simulink model "Model_14Bus_Microgrid_paper_Latam"  (R2022b)
settings: Solver=VariableStepAuto  StartTime=0.0  StopTime=0.5  MaxStep=1e-2  RelTol=1e-3
InitFcn:
  | Set_parameters_R2018
StopFcn:
  | %Save_Data;
  | %Graphics_mod;
values from neighbouring files (symbols this model uses):
  Clink = Ceq*2    (= 0.217013888889)    [Set_parameters.m]
  dis1 = 0.15    [Set_parameters.m]
  dis10 = 6    [Set_parameters.m]
  dis11 = 3    [Set_parameters.m]
  dis12 = 6    [Set_parameters.m]
  dis13 = 3    [Set_parameters.m]
  dis14 = 2    [Set_parameters.m]
  dis2 = 0.2    [Set_parameters.m]
  dis3 = 0.15    [Set_parameters.m]
  dis4 = 0.4    [Set_parameters.m]
  dis5 = 0.4    [Set_parameters.m]
  dis6 = 0.4    [Set_parameters.m]
  dis7 = 0.1    [Set_parameters.m]
  dis8 = 2    [Set_parameters.m]
  dis9 = 6    [Set_parameters.m]
  Fc = 33 * Fnom    (= 1980)    [Set_parameters.m]
  Fnom = 60    [Set_parameters.m]
  Increment_MPPT = 0.01    [Set_parameters.m]
  Ki_Ireg = 20    [Set_parameters.m]
  Ki_VDCreg = 400    [Set_parameters.m]
  Kp_Ireg = 0.3    [Set_parameters.m]
  Kp_VDCreg = 2    [Set_parameters.m]
  LimitL_Ireg = -1.5    [Set_parameters.m]
  LimitL_VDCreg = -1.5    [Set_parameters.m]
  Limits_MPPT = [ 583 357 ]    [Set_parameters.m]
  LimitU_Ireg = 1.5    [Set_parameters.m]
  LimitU_VDCreg = 1.5    [Set_parameters.m]
  P_Load_2 = S_Load_2* PF_Load_2    (= 36000)    [Set_parameters.m]
  P_Load_3 = S_Load_3* PF_Load_3    (= 25500)    [Set_parameters.m]
  Pnom = 1e6    (= 1000000)    [Set_parameters.m]
  Pnom_T1 = 1.5e6    (= 1500000)    [Set_parameters.m]
  Pnom_T2 = 1.5e6    (= 1500000)    [Set_parameters.m]
  Pnom_T3 = 4e6    (= 4000000)    [Set_parameters.m]
  Pnom_xfo = Pnom    (= 1000000)    [Set_parameters.m]
  Ql_Load_2 = S_Load_2 * sin(acos(PF_Load_2))    [Set_parameters.m]
  Ql_Load_3 = S_Load_3 * sin(acos(PF_Load_3))    [Set_parameters.m]
  R_Load_9 = (Vnom_prim * 1.35)^2 / P_Load_9    (= 1084.6153125)    [Set_parameters.m]
  R_Load_DC = Vnom_DC^2/ P_Load_DC    (= 45)    [Set_parameters.m]
  Rl = 0.394    [Set_parameters.m]
  Rls = 0.198    [Set_parameters.m]
  Ts = Ts_Power    (= 5.05050505051e-06)    [Set_parameters.m]
  Ts_Control = 10*Ts_Power    (= 5.05050505051e-05)    [Set_parameters.m]
  Ts_Power = 1/(33*Fnom)/100    (= 5.05050505051e-06)    [Set_parameters.m]
  V1_LL_T3 = 69e3    (= 69000)    [Set_parameters.m]
  Vf = 0    [Set_parameters.m]
  Vfd = 0    [Set_parameters.m]
  Vnom_dc = 480    [Set_parameters.m]
  Vnom_Diesel = 2.4e3    (= 2400)    [Set_parameters.m]
  Vnom_prim = 13.8e3    (= 13800)    [Set_parameters.m]
  Vnom_sec = 220    [Set_parameters.m]
  Vnom_ter_AC_DC = 150    [Set_parameters.m]
  Xl = 0.1168    [Set_parameters.m]
  Xls = 0.1089    [Set_parameters.m]
undefined symbols (not defined in the file or in its folder): D1, Delta, DiscIntNeverNeededParam, Hydride, Ion, level, Lithium, max_min, Metal, Nickel, RL, RLff, sigbuilder_block
libraries: spsRMSLib x73, powerlib_extras x53, spsCurrentMeasurementLib x47, spsTHDLib x26, spsThreePhaseVIMeasurementLib x25, spsVoltageMeasurementLib x23, spsSeriesRLCBranchLib x21, spsThreePhaseSeriesRLCBranchLib x21, spsIGBTDiodeLib x15, spsThreePhaseBreakerLib x14, spsPowerLib x14, spsThreePhaseTransformerTwoWindingsLib x12
(part 3 of 10)

== system Model_14Bus_Microgrid_paper_Latam/Line 10 (6km) ==
  Bus_14 11 : Subsystem  Commented=on
  Goto30 : Goto  Commented=on  GotoTag=Ib_L10  TagVisibility=global
  Goto31 : Goto  Commented=on  GotoTag=Ic_L10  TagVisibility=global
  Goto32 : Goto  Commented=on  GotoTag=Ia_L10  TagVisibility=global
  Ia_L10 : spsCurrentMeasurementLib/Current Measurement  PhasorSimulation=off  OutputType=Complex  PSBequivalent=0
  Ib_L10 : spsCurrentMeasurementLib/Current Measurement  PhasorSimulation=off  OutputType=Complex  PSBequivalent=0
  Ic_L10 : spsCurrentMeasurementLib/Current Measurement  PhasorSimulation=off  OutputType=Complex  PSBequivalent=0
  Line10 6km : spsThreePhaseSeriesRLCBranchLib/Three-Phase Series RLC Branch  LConnTagsString=A|B|C  RConnTagsString=A|B|C  BranchType=RL  Resistance=Rl * dis10  Inductance=Xl/377 * dis10  Capacitance=1e-6  Measurements=None
  a : PMIOPort  Side=Right
  b : PMIOPort  Port=2  Side=Right
  c : PMIOPort  Port=3  Side=Right
  A : PMIOPort  Port=4  Side=Left
  B : PMIOPort  Port=5  Side=Left
  C : PMIOPort  Port=6  Side=Left
  wires:
  Ia_L10/1 -> Goto32/1
  Ic_L10/1 -> Goto31/1
  Ib_L10/1 -> Goto30/1
  connections:
  B/RConn1 -- Line10 6km/LConn2
  b/RConn1 -- Ib_L10/RConn1
  Line10 6km/RConn2 -- Ib_L10/LConn1
  C/RConn1 -- Line10 6km/LConn3
  c/RConn1 -- Ic_L10/RConn1
  Line10 6km/RConn1 -- Ia_L10/LConn1
  Line10 6km/RConn3 -- Ic_L10/LConn1
  A/RConn1 -- Line10 6km/LConn1
  a/RConn1 -- Ia_L10/RConn1

== system Model_14Bus_Microgrid_paper_Latam/Line 11 (3 km) ==
  "  Ic_L11" : spsCurrentMeasurementLib/Current Measurement  PhasorSimulation=off  OutputType=Complex  PSBequivalent=0
  Bus_14 12 : Subsystem  Commented=on
  Goto33 : Goto  Commented=on  GotoTag=Ib_L11  TagVisibility=global
  Goto34 : Goto  Commented=on  GotoTag=Ic_L11  TagVisibility=global
  Goto35 : Goto  Commented=on  GotoTag=Ia_L11  TagVisibility=global
  Ia_L11 : spsCurrentMeasurementLib/Current Measurement  PhasorSimulation=off  OutputType=Complex  PSBequivalent=0
  Ib_L11 : spsCurrentMeasurementLib/Current Measurement  PhasorSimulation=off  OutputType=Complex  PSBequivalent=0
  Line11 3km : spsThreePhaseSeriesRLCBranchLib/Three-Phase Series RLC Branch  LConnTagsString=A|B|C  RConnTagsString=A|B|C  BranchType=RL  Resistance=Rl* dis11  Inductance=Xl/377 * dis11  Capacitance=1e-6  Measurements=None
  a : PMIOPort  Side=Left
  b : PMIOPort  Port=2  Side=Left
  c : PMIOPort  Port=3  Side=Left
  C : PMIOPort  Port=4  Side=Right
  B : PMIOPort  Port=5  Side=Right
  A : PMIOPort  Port=6  Side=Right
  wires:
  Ia_L11/1 -> Goto35/1
  Ib_L11/1 -> Goto33/1
  "  Ic_L11"/1 -> Goto34/1
  connections:
  B/RConn1 -- Line11 3km/LConn2
  Line11 3km/LConn3 -- C/RConn1
  Ia_L11/LConn1 -- a/RConn1
  Line11 3km/RConn1 -- Ia_L11/RConn1
  Line11 3km/RConn3 -- "  Ic_L11"/RConn1
  Line11 3km/RConn2 -- Ib_L11/RConn1
  c/RConn1 -- "  Ic_L11"/LConn1
  Line11 3km/LConn1 -- A/RConn1
  Ib_L11/LConn1 -- b/RConn1

== system Model_14Bus_Microgrid_paper_Latam/Line 12 (6km) ==
  Bus_14 13 : Subsystem  Commented=on
  Goto36 : Goto  Commented=on  GotoTag=Ia_L12  TagVisibility=global
  Goto37 : Goto  Commented=on  GotoTag=Ib_L12  TagVisibility=global
  Goto38 : Goto  Commented=on  GotoTag=Ic_L12  TagVisibility=global
  Ia_L12 : spsCurrentMeasurementLib/Current Measurement  PhasorSimulation=off  OutputType=Complex  PSBequivalent=0
  Ib_L12 : spsCurrentMeasurementLib/Current Measurement  PhasorSimulation=off  OutputType=Complex  PSBequivalent=0
  Ic_L12 : spsCurrentMeasurementLib/Current Measurement  PhasorSimulation=off  OutputType=Complex  PSBequivalent=0
  Line12 6km : spsThreePhaseSeriesRLCBranchLib/Three-Phase Series RLC Branch  LConnTagsString=A|B|C  RConnTagsString=A|B|C  BranchType=RL  Resistance=Rl * dis12  Inductance=Xl/377 * dis12  Capacitance=1e-6  Measurements=None
  C : PMIOPort  Side=Left
  B : PMIOPort  Port=2  Side=Left
  A : PMIOPort  Port=3  Side=Left
  a : PMIOPort  Port=4  Side=Right
  b : PMIOPort  Port=5  Side=Right
  c : PMIOPort  Port=6  Side=Right
  wires:
  Ib_L12/1 -> Goto37/1
  Ia_L12/1 -> Goto36/1
  Ic_L12/1 -> Goto38/1
  connections:
  C/RConn1 -- Ic_L12/LConn1
  Line12 6km/RConn1 -- a/RConn1
  Ia_L12/LConn1 -- A/RConn1
  Line12 6km/LConn1 -- Ia_L12/RConn1
  Line12 6km/RConn3 -- c/RConn1
  Ib_L12/LConn1 -- B/RConn1
  Line12 6km/LConn2 -- Ib_L12/RConn1
  Line12 6km/RConn2 -- b/RConn1
  Line12 6km/LConn3 -- Ic_L12/RConn1

== system Model_14Bus_Microgrid_paper_Latam/Line 13 (3km) ==
  Bus14_1 : spsThreePhaseVIMeasurementLib/Three-Phase V-I Measurement  VoltageMeasurement=phase-to-ground  SetLabelV=on  LabelV=Vabc_load_14_1  Vpu=off  VpuLL=off  CurrentMeasurement=yes  SetLabelI=on  LabelI=Iabc_load_14_1  Ipu=off  Pbase=100e6  Vbase=380/sqrt(2)  OutputType=Complex  PhasorSimulation=off  PSBequivalent=0
  Bus_14 1 : Subsystem  Commented=on
  Goto : Goto  Commented=on  GotoTag=Ia_L13  TagVisibility=global
  Goto1 : Goto  Commented=on  GotoTag=Ib_L13  TagVisibility=global
  Goto2 : Goto  Commented=on  GotoTag=Ic_L13  TagVisibility=global
  Ia_L13 : spsCurrentMeasurementLib/Current Measurement  PhasorSimulation=off  OutputType=Complex  PSBequivalent=0
  Ib_L13 : spsCurrentMeasurementLib/Current Measurement  PhasorSimulation=off  OutputType=Complex  PSBequivalent=0
  Ic_L13 : spsCurrentMeasurementLib/Current Measurement  PhasorSimulation=off  OutputType=Complex  PSBequivalent=0
  Line13 3km : spsThreePhaseSeriesRLCBranchLib/Three-Phase Series RLC Branch  LConnTagsString=A|B|C  RConnTagsString=A|B|C  BranchType=RL  Resistance=Rl * dis13  Inductance=Xl/377 * dis13  Capacitance=1e-6  Measurements=None
  Load_4 : Subsystem
      mask Display: image('/Users/christian/Documents/MATLAB/doctorado/4 conectada a la red con generador diesel, con generacion renovanble (fv)-con almacenamiento varios scope/Icons/S_meeter.png'); % Use "Edit Image" on toolstrip to change.
  A : PMIOPort  Side=Left
  a : PMIOPort  Port=2  Side=Right
  B : PMIOPort  Port=3  Side=Left
  b : PMIOPort  Port=4  Side=Right
  C : PMIOPort  Port=5  Side=Left
  c : PMIOPort  Port=6  Side=Right
  wires:
  Ib_L13/1 -> Goto1/1
  Ic_L13/1 -> Goto2/1
  Ia_L13/1 -> Goto/1
  connections:
  Bus14_1/RConn2 -- b/RConn1
  Bus14_1/RConn3 -- c/RConn1
  Line13 3km/RConn3 -- Ic_L13/LConn1
  Bus14_1/LConn3 -- Ic_L13/RConn1
  Line13 3km/LConn2 -- B/RConn1
  Bus14_1/RConn1 -- a/RConn1
  Line13 3km/RConn2 -- Ib_L13/LConn1
  Bus14_1/LConn1 -- Ia_L13/RConn1
  Line13 3km/LConn1 -- A/RConn1
  Bus14_1/LConn2 -- Ib_L13/RConn1
  Line13 3km/RConn1 -- Ia_L13/LConn1
  Line13 3km/LConn3 -- C/RConn1

== system Model_14Bus_Microgrid_paper_Latam/Line 2 (200m) ==
  Bus_14 2 : Subsystem  Commented=on
  Goto3 : Goto  Commented=on  GotoTag=Ia_L2  TagVisibility=global
  Goto4 : Goto  Commented=on  GotoTag=Ib_L2  TagVisibility=global
  Goto5 : Goto  Commented=on  GotoTag=Ic_L2  TagVisibility=global
  Ia_L2 : spsCurrentMeasurementLib/Current Measurement  PhasorSimulation=off  OutputType=Complex  PSBequivalent=0
  Ib_L2 : spsCurrentMeasurementLib/Current Measurement  PhasorSimulation=off  OutputType=Complex  PSBequivalent=0
  Ic_L2 : spsCurrentMeasurementLib/Current Measurement  PhasorSimulation=off  OutputType=Complex  PSBequivalent=0
  Line2 200m : spsThreePhaseSeriesRLCBranchLib/Three-Phase Series RLC Branch  LConnTagsString=A|B|C  RConnTagsString=A|B|C  BranchType=RL  Resistance=Rls * dis2  Inductance=Xls/377 * dis2  Capacitance=1e-6  Measurements=None
  A : PMIOPort  Side=Left
  B : PMIOPort  Port=2  Side=Left
  C : PMIOPort  Port=3  Side=Left
  a : PMIOPort  Port=4  Side=Right
  b : PMIOPort  Port=5  Side=Right
  c : PMIOPort  Port=6  Side=Right
  wires:
  Ib_L2/1 -> Goto4/1
  Ic_L2/1 -> Goto5/1
  Ia_L2/1 -> Goto3/1
  connections:
  b/RConn1 -- Line2 200m/RConn2
  Line2 200m/RConn3 -- c/RConn1
  Ib_L2/RConn1 -- B/RConn1
  Line2 200m/LConn2 -- Ib_L2/LConn1
  Line2 200m/LConn1 -- Ia_L2/LConn1
  Ic_L2/RConn1 -- C/RConn1
  Ia_L2/RConn1 -- A/RConn1
  Line2 200m/RConn1 -- a/RConn1
  Line2 200m/LConn3 -- Ic_L2/LConn1

== system Model_14Bus_Microgrid_paper_Latam/Line 3 (150m) ==
  "  Ic_L3" : spsCurrentMeasurementLib/Current Measurement  PhasorSimulation=off  OutputType=Complex  PSBequivalent=0
  Bus_14 7 : Subsystem  Commented=on
  Goto18 : Goto  Commented=on  GotoTag=Ib_L3  TagVisibility=global
  Goto19 : Goto  Commented=on  GotoTag=Ic_L3  TagVisibility=global
  Goto20 : Goto  Commented=on  GotoTag=Ia_L3  TagVisibility=global
  Ia_L3 : spsCurrentMeasurementLib/Current Measurement  PhasorSimulation=off  OutputType=Complex  PSBequivalent=0
  Ib_L3 : spsCurrentMeasurementLib/Current Measurement  PhasorSimulation=off  OutputType=Complex  PSBequivalent=0
  Line3 150m : spsThreePhaseSeriesRLCBranchLib/Three-Phase Series RLC Branch  LConnTagsString=A|B|C  RConnTagsString=A|B|C  BranchType=RL  Resistance=Rls * dis3  Inductance=Xls/377 * dis3  Capacitance=1e-6  Measurements=None
  a : PMIOPort  Side=Left
  b : PMIOPort  Port=2  Side=Left
  c : PMIOPort  Port=3  Side=Left
  A : PMIOPort  Port=4  Side=Right
  B : PMIOPort  Port=5  Side=Right
  C : PMIOPort  Port=6  Side=Right
  wires:
  "  Ic_L3"/1 -> Goto19/1
  Ia_L3/1 -> Goto20/1
  Ib_L3/1 -> Goto18/1
  connections:
  Ib_L3/LConn1 -- b/RConn1
  "  Ic_L3"/LConn1 -- c/RConn1
  Ia_L3/LConn1 -- a/RConn1
  Line3 150m/RConn3 -- "  Ic_L3"/RConn1
  Line3 150m/RConn1 -- Ia_L3/RConn1
  Line3 150m/LConn2 -- B/RConn1
  Line3 150m/LConn3 -- C/RConn1
  Line3 150m/LConn1 -- A/RConn1
  Line3 150m/RConn2 -- Ib_L3/RConn1

== system Model_14Bus_Microgrid_paper_Latam/Line 4 (400m) ==
  "  Ic_L4" : spsCurrentMeasurementLib/Current Measurement  PhasorSimulation=off  OutputType=Complex  PSBequivalent=0
  Bus_14 6 : Subsystem  Commented=on
  Goto15 : Goto  Commented=on  GotoTag=Ib_L4  TagVisibility=global
  Goto16 : Goto  Commented=on  GotoTag=Ic_L4  TagVisibility=global
  Goto17 : Goto  Commented=on  GotoTag=Ia_L4  TagVisibility=global
  Ia_L4 : spsCurrentMeasurementLib/Current Measurement  PhasorSimulation=off  OutputType=Complex  PSBequivalent=0
  Ib_L4 : spsCurrentMeasurementLib/Current Measurement  PhasorSimulation=off  OutputType=Complex  PSBequivalent=0
  Line4 400m : spsThreePhaseSeriesRLCBranchLib/Three-Phase Series RLC Branch  LConnTagsString=A|B|C  RConnTagsString=A|B|C  BranchType=RL  Resistance=Rls * dis4  Inductance=Xls/377 * dis4  Capacitance=1e-6  Measurements=None
  a : PMIOPort  Side=Left
  b : PMIOPort  Port=2  Side=Left
  c : PMIOPort  Port=3  Side=Left
  C : PMIOPort  Port=6  Side=Right
  A : PMIOPort  Port=4  Side=Right
  B : PMIOPort  Port=5  Side=Right
  wires:
  "  Ic_L4"/1 -> Goto16/1
  Ia_L4/1 -> Goto17/1
  Ib_L4/1 -> Goto15/1
  connections:
  c/RConn1 -- "  Ic_L4"/LConn1
  Line4 400m/RConn1 -- Ia_L4/RConn1
  A/RConn1 -- Line4 400m/LConn1
  Ib_L4/LConn1 -- b/RConn1
  B/RConn1 -- Line4 400m/LConn2
  Line4 400m/RConn2 -- Ib_L4/RConn1
  C/RConn1 -- Line4 400m/LConn3
  Line4 400m/RConn3 -- "  Ic_L4"/RConn1
  Ia_L4/LConn1 -- a/RConn1

== system Model_14Bus_Microgrid_paper_Latam/Line 5 (400m) ==
  Bus_14 5 : Subsystem  Commented=on
  Goto12 : Goto  Commented=on  GotoTag=Ib_L5  TagVisibility=global
  Goto13 : Goto  Commented=on  GotoTag=Ic_L5  TagVisibility=global
  Goto14 : Goto  Commented=on  GotoTag=Ia_L5  TagVisibility=global
  Ia_L5 : spsCurrentMeasurementLib/Current Measurement  PhasorSimulation=off  OutputType=Complex  PSBequivalent=0
  Ib_L5 : spsCurrentMeasurementLib/Current Measurement  PhasorSimulation=off  OutputType=Complex  PSBequivalent=0
  Ic_L5 : spsCurrentMeasurementLib/Current Measurement  PhasorSimulation=off  OutputType=Complex  PSBequivalent=0
  Line5 400m : spsThreePhaseSeriesRLCBranchLib/Three-Phase Series RLC Branch  LConnTagsString=A|B|C  RConnTagsString=A|B|C  BranchType=RL  Resistance=Rls * dis5  Inductance=Xls/377 * dis5  Capacitance=1e-6  Measurements=None
  a : PMIOPort  Side=Right
  A : PMIOPort  Port=2  Side=Left
  B : PMIOPort  Port=3  Side=Left
  b : PMIOPort  Port=4  Side=Right
  C : PMIOPort  Port=5  Side=Left
  c : PMIOPort  Port=6  Side=Right
  wires:
  Ib_L5/1 -> Goto12/1
  Ic_L5/1 -> Goto13/1
  Ia_L5/1 -> Goto14/1
  connections:
  Line5 400m/LConn2 -- B/RConn1
  Line5 400m/RConn1 -- Ia_L5/LConn1
  Line5 400m/LConn1 -- A/RConn1
  Line5 400m/LConn3 -- C/RConn1
  Ib_L5/RConn1 -- b/RConn1
  Ic_L5/RConn1 -- c/RConn1
  Ia_L5/RConn1 -- a/RConn1
  Line5 400m/RConn2 -- Ib_L5/LConn1
  Line5 400m/RConn3 -- Ic_L5/LConn1

== system Model_14Bus_Microgrid_paper_Latam/Line 6 (400m) ==
  Bus_14 4 : Subsystem  Commented=on
  Goto10 : Goto  Commented=on  GotoTag=Ib_L6  TagVisibility=global
  Goto11 : Goto  Commented=on  GotoTag=Ic_L6  TagVisibility=global
  Goto9 : Goto  Commented=on  GotoTag=Ia_L6  TagVisibility=global
  Ia_L6 : spsCurrentMeasurementLib/Current Measurement  PhasorSimulation=off  OutputType=Complex  PSBequivalent=0
  Ib_L6 : spsCurrentMeasurementLib/Current Measurement  PhasorSimulation=off  OutputType=Complex  PSBequivalent=0
  Ic_L6 : spsCurrentMeasurementLib/Current Measurement  PhasorSimulation=off  OutputType=Complex  PSBequivalent=0
  Line6 400m : spsThreePhaseSeriesRLCBranchLib/Three-Phase Series RLC Branch  LConnTagsString=A|B|C  RConnTagsString=A|B|C  BranchType=RL  Resistance=Rls * dis6  Inductance=Xls/377 * dis6  Capacitance=1e-6  Measurements=None
  A : PMIOPort  Side=Left
  a : PMIOPort  Port=2  Side=Right
  B : PMIOPort  Port=3  Side=Left
  b : PMIOPort  Port=4  Side=Right
  C : PMIOPort  Port=5  Side=Left
  c : PMIOPort  Port=6  Side=Right
  wires:
  Ia_L6/1 -> Goto9/1
  Ib_L6/1 -> Goto10/1
  Ic_L6/1 -> Goto11/1
  connections:
  Line6 400m/LConn2 -- B/RConn1
  b/RConn1 -- Ib_L6/RConn1
  a/RConn1 -- Ia_L6/RConn1
  Line6 400m/LConn3 -- C/RConn1
  Line6 400m/RConn1 -- Ia_L6/LConn1
  Line6 400m/LConn1 -- A/RConn1
  c/RConn1 -- Ic_L6/RConn1
  Line6 400m/RConn3 -- Ic_L6/LConn1
  Line6 400m/RConn2 -- Ib_L6/LConn1

== system Model_14Bus_Microgrid_paper_Latam/Line 7 (100m) ==
  "  Ic_L7" : spsCurrentMeasurementLib/Current Measurement  PhasorSimulation=off  OutputType=Complex  PSBequivalent=0
  Bus_14 8 : Subsystem  Commented=on
  Goto21 : Goto  Commented=on  GotoTag=Ib_L7  TagVisibility=global
  Goto22 : Goto  Commented=on  GotoTag=Ic_L7  TagVisibility=global
  Goto23 : Goto  Commented=on  GotoTag=Ia_L7  TagVisibility=global
  Ia_L7 : spsCurrentMeasurementLib/Current Measurement  PhasorSimulation=off  OutputType=Complex  PSBequivalent=0
  Ib_L7 : spsCurrentMeasurementLib/Current Measurement  PhasorSimulation=off  OutputType=Complex  PSBequivalent=0
  Line7 100m : spsThreePhaseSeriesRLCBranchLib/Three-Phase Series RLC Branch  LConnTagsString=A|B|C  RConnTagsString=A|B|C  BranchType=RL  Resistance=Rls * dis7  Inductance=Xls/377 * dis7  Capacitance=1e-6  Measurements=None
  a : PMIOPort  Side=Left
  b : PMIOPort  Port=2  Side=Left
  c : PMIOPort  Port=3  Side=Left
  A : PMIOPort  Port=4  Side=Right
  B : PMIOPort  Port=5  Side=Right
  C : PMIOPort  Port=6  Side=Right
  wires:
  Ia_L7/1 -> Goto23/1
  Ib_L7/1 -> Goto21/1
  "  Ic_L7"/1 -> Goto22/1
  connections:
  B/RConn1 -- Line7 100m/LConn2
  "  Ic_L7"/LConn1 -- c/RConn1
  Line7 100m/RConn2 -- Ib_L7/RConn1
  C/RConn1 -- Line7 100m/LConn3
  Line7 100m/RConn1 -- Ia_L7/RConn1
  A/RConn1 -- Line7 100m/LConn1
  Line7 100m/RConn3 -- "  Ic_L7"/RConn1
  Ia_L7/LConn1 -- a/RConn1
  Ib_L7/LConn1 -- b/RConn1

== system Model_14Bus_Microgrid_paper_Latam/Line 8 (2km)  ==
  "  Ic_L8" : spsCurrentMeasurementLib/Current Measurement  PhasorSimulation=off  OutputType=Complex  PSBequivalent=0
  Bus_14 9 : Subsystem  Commented=on
  Goto24 : Goto  Commented=on  GotoTag=Ib_L8  TagVisibility=global
  Goto25 : Goto  Commented=on  GotoTag=Ic_L8  TagVisibility=global
  Goto26 : Goto  Commented=on  GotoTag=Ia_L8  TagVisibility=global
  Ia_L8 : spsCurrentMeasurementLib/Current Measurement  PhasorSimulation=off  OutputType=Complex  PSBequivalent=0
  Ib_L8 : spsCurrentMeasurementLib/Current Measurement  PhasorSimulation=off  OutputType=Complex  PSBequivalent=0
  Line8 2km : spsThreePhaseSeriesRLCBranchLib/Three-Phase Series RLC Branch  LConnTagsString=A|B|C  RConnTagsString=A|B|C  BranchType=RL  Resistance=Rl * dis8  Inductance=Xl/377 * dis8  Capacitance=1e-6  Measurements=None
  a : PMIOPort  Side=Left
  b : PMIOPort  Port=2  Side=Left
  c : PMIOPort  Port=3  Side=Left
  A : PMIOPort  Port=4  Side=Right
  B : PMIOPort  Port=5  Side=Right
  C : PMIOPort  Port=6  Side=Right
  wires:
  "  Ic_L8"/1 -> Goto25/1
  Ia_L8/1 -> Goto26/1
  Ib_L8/1 -> Goto24/1
  connections:
  C/RConn1 -- Line8 2km/LConn3
  A/RConn1 -- Line8 2km/LConn1
  b/RConn1 -- Ib_L8/LConn1
  B/RConn1 -- Line8 2km/LConn2
  Line8 2km/RConn2 -- Ib_L8/RConn1
  c/RConn1 -- "  Ic_L8"/LConn1
  Line8 2km/RConn3 -- "  Ic_L8"/RConn1
  Line8 2km/RConn1 -- Ia_L8/RConn1
  a/RConn1 -- Ia_L8/LConn1

== system Model_14Bus_Microgrid_paper_Latam/Line 9 (6km) ==
  "  Ic_L9" : spsCurrentMeasurementLib/Current Measurement  PhasorSimulation=off  OutputType=Complex  PSBequivalent=0
  Bus_14 10 : Subsystem  Commented=on
  Goto27 : Goto  Commented=on  GotoTag=Ib_L9  TagVisibility=global
  Goto28 : Goto  Commented=on  GotoTag=Ic_L9  TagVisibility=global
  Goto29 : Goto  Commented=on  GotoTag=Ia_L9  TagVisibility=global
  Ia_L9 : spsCurrentMeasurementLib/Current Measurement  PhasorSimulation=off  OutputType=Complex  PSBequivalent=0
  Ib_L9 : spsCurrentMeasurementLib/Current Measurement  PhasorSimulation=off  OutputType=Complex  PSBequivalent=0
  Line9 6km : spsThreePhaseSeriesRLCBranchLib/Three-Phase Series RLC Branch  LConnTagsString=A|B|C  RConnTagsString=A|B|C  BranchType=RL  Resistance=Rl * dis9  Inductance=Xl/377 * dis9  Capacitance=1e-6  Measurements=None
  a : PMIOPort  Side=Left
  b : PMIOPort  Port=2  Side=Left
  c : PMIOPort  Port=3  Side=Left
  A : PMIOPort  Port=4  Side=Right
  B : PMIOPort  Port=5  Side=Right
  C : PMIOPort  Port=6  Side=Right
  wires:
  Ib_L9/1 -> Goto27/1
  Ia_L9/1 -> Goto29/1
  "  Ic_L9"/1 -> Goto28/1
  connections:
  a/RConn1 -- Ia_L9/LConn1
  Ib_L9/LConn1 -- b/RConn1
  "  Ic_L9"/LConn1 -- c/RConn1
  Line9 6km/LConn1 -- A/RConn1
  Line9 6km/LConn3 -- C/RConn1
  Line9 6km/RConn3 -- "  Ic_L9"/RConn1
  Line9 6km/RConn1 -- Ia_L9/RConn1
  Line9 6km/LConn2 -- B/RConn1
  Line9 6km/RConn2 -- Ib_L9/RConn1

== system Model_14Bus_Microgrid_paper_Latam/Line14 (2km) ==
  Bus_14 14 : Subsystem  Commented=on
  Goto39 : Goto  Commented=on  GotoTag=Ib_L14  TagVisibility=global
  Goto40 : Goto  Commented=on  GotoTag=Ic_L14  TagVisibility=global
  Goto41 : Goto  Commented=on  GotoTag=Ia_L14  TagVisibility=global
  Ia_L14 : spsCurrentMeasurementLib/Current Measurement  PhasorSimulation=off  OutputType=Complex  PSBequivalent=0
  Ib_L14 : spsCurrentMeasurementLib/Current Measurement  PhasorSimulation=off  OutputType=Complex  PSBequivalent=0
  Ic_L14 : spsCurrentMeasurementLib/Current Measurement  PhasorSimulation=off  OutputType=Complex  PSBequivalent=0
  Line14 2km : spsThreePhaseSeriesRLCBranchLib/Three-Phase Series RLC Branch  LConnTagsString=A|B|C  RConnTagsString=A|B|C  BranchType=RL  Resistance=Rl * dis14  Inductance=Xl/377 * dis14  Capacitance=1e-6  Measurements=None
  a : PMIOPort  Side=Left
  b : PMIOPort  Port=2  Side=Left
  c : PMIOPort  Port=3  Side=Left
  A : PMIOPort  Port=4  Side=Right
  B : PMIOPort  Port=5  Side=Right
  C : PMIOPort  Port=6  Side=Right
  wires:
  Ib_L14/1 -> Goto39/1
  Ic_L14/1 -> Goto40/1
  Ia_L14/1 -> Goto41/1
  connections:
  Line14 2km/LConn3 -- C/RConn1
  Ic_L14/LConn1 -- c/RConn1
  Ia_L14/LConn1 -- a/RConn1
  Line14 2km/LConn2 -- B/RConn1
  Line14 2km/RConn3 -- Ic_L14/RConn1
  Line14 2km/LConn1 -- A/RConn1
  Ib_L14/LConn1 -- b/RConn1
  Line14 2km/RConn2 -- Ib_L14/RConn1
  Line14 2km/RConn1 -- Ia_L14/RConn1

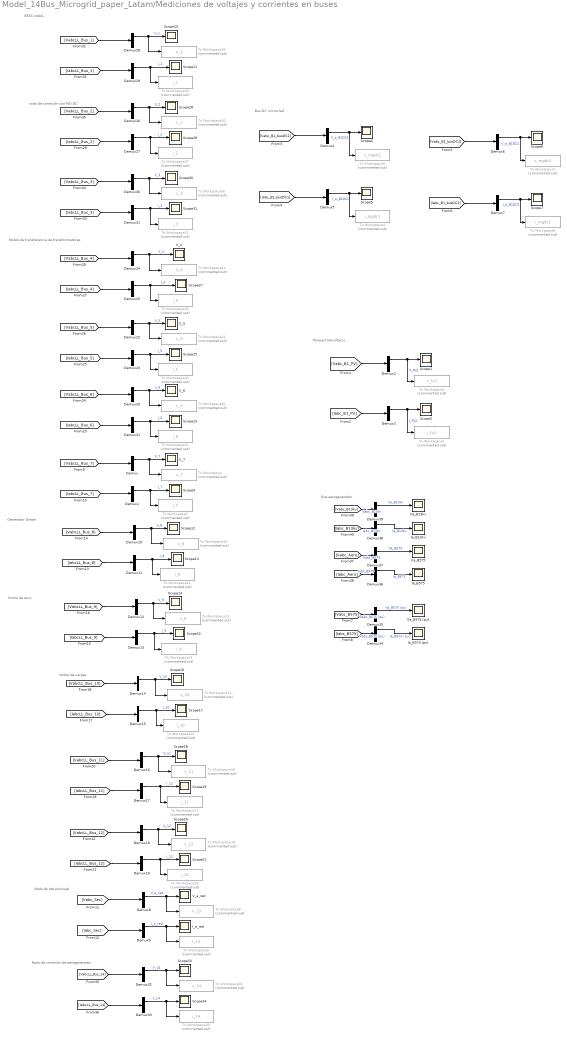
== system Model_14Bus_Microgrid_paper_Latam/Mediciones de voltajes y corrientes en buses ==
  note: Nodos de cargas
  note: Nodo de conexión de aerogenerador
  note: Nodo de red principal
  note: Horno de arco
  note: Generador Diesel
  note: nodo de conexión con MG DC
  note: BESS nodo1
  note: Parque fotovoltaico
  note: Bus DC microrred
  note: Nodos de transferencia de transformadores
  note: Bus aerogenerador
  Demux{,1..39} (40 alike) : Demux  Outputs=3
  I_a_red : Scope
  Ia_B13kv : Scope
  Ia_B575 : Scope
  Ia_B575 (pu) : Scope
  Scope{1..2,4..7,9..21,23,25,27..31,33..34} (28 alike) : Scope
  To Workspace : ToWorkspace  Commented=on  VariableName=v_7  SampleTime=-1
  To Workspace1 : ToWorkspace  Commented=on  VariableName=i_7  SampleTime=-1
  To Workspace10 : ToWorkspace  Commented=on  VariableName=v_8  SampleTime=-1
  To Workspace11 : ToWorkspace  Commented=on  VariableName=i_8  SampleTime=-1
  To Workspace12 : ToWorkspace  Commented=on  VariableName=v_9  SampleTime=-1
  To Workspace13 : ToWorkspace  Commented=on  VariableName=i_9  SampleTime=-1
  To Workspace14 : ToWorkspace  Commented=on  VariableName=v_10  SampleTime=-1
  To Workspace15 : ToWorkspace  Commented=on  VariableName=i_10  SampleTime=-1
  To Workspace16 : ToWorkspace  Commented=on  VariableName=v_11  SampleTime=-1
  To Workspace17 : ToWorkspace  Commented=on  VariableName=i_11  SampleTime=-1
  To Workspace18 : ToWorkspace  Commented=on  VariableName=v_12  SampleTime=-1
  To Workspace19 : ToWorkspace  Commented=on  VariableName=i_12  SampleTime=-1
  To Workspace2 : ToWorkspace  Commented=on  VariableName=v_fv2  SampleTime=-1
  To Workspace20 : ToWorkspace  Commented=on  VariableName=v_6  SampleTime=-1
  To Workspace21 : ToWorkspace  Commented=on  VariableName=i_6  SampleTime=-1
  To Workspace22 : ToWorkspace  Commented=on  VariableName=v_5  SampleTime=-1
  To Workspace23 : ToWorkspace  Commented=on  VariableName=i_5  SampleTime=-1
  To Workspace24 : ToWorkspace  Commented=on  VariableName=v_4  SampleTime=-1
  To Workspace25 : ToWorkspace  Commented=on  VariableName=i_4  SampleTime=-1
  To Workspace26 : ToWorkspace  Commented=on  VariableName=v_2  SampleTime=-1
  To Workspace27 : ToWorkspace  Commented=on  VariableName=i_2  SampleTime=-1
  To Workspace28 : ToWorkspace  Commented=on  VariableName=v_1  SampleTime=-1
  To Workspace29 : ToWorkspace  Commented=on  VariableName=i_1  SampleTime=-1
  To Workspace3 : ToWorkspace  Commented=on  VariableName=i_fv2  SampleTime=-1
  To Workspace30 : ToWorkspace  Commented=on  VariableName=v_3  SampleTime=-1
  To Workspace31 : ToWorkspace  Commented=on  VariableName=i_3  SampleTime=-1
  To Workspace32 : ToWorkspace  Commented=on  VariableName=v_14  SampleTime=-1
  To Workspace33 : ToWorkspace  Commented=on  VariableName=i_14  SampleTime=-1
  To Workspace4 : ToWorkspace  Commented=on  VariableName=i_mgdc1  SampleTime=-1
  To Workspace5 : ToWorkspace  Commented=on  VariableName=v_mgdc1  SampleTime=-1
  To Workspace6 : ToWorkspace  Commented=on  VariableName=i_mgdc2  SampleTime=-1
  To Workspace7 : ToWorkspace  Commented=on  VariableName=v_mgdc2  SampleTime=-1
  To Workspace8 : ToWorkspace  Commented=on  VariableName=v_13  SampleTime=-1
  To Workspace9 : ToWorkspace  Commented=on  VariableName=i_13  SampleTime=-1
  V_{4..7} (4 alike) : Scope
  V_a_red : Scope
  Va_B13kv : Scope
  Va_B575 : Scope
  Va_B575 (pu) : Scope
  wires:
  [VabcLL_Bus_7] -> Demux/1
  Demux12/1 -> Scope14/1, To Workspace12/1  "V_9"
  [VabcLL_Bus_1] -> Demux28/1
  Demux7/1 -> Scope7/1, To Workspace6/1  "I_a_B1DC2"
  [Vabc_B1_busDC1] -> Demux4/1
  [VabcLL_Bus_3] -> Demux30/1
  [Vabc_B1_busDC2] -> Demux6/1
  [IabcLL_Bus_10] -> Demux15/1
  [IabcLL_Bus_12] -> Demux19/1
  Demux18/1 -> Scope20/1, To Workspace18/1  "V_12"
  Demux2/1 -> Scope1/1, To Workspace2/1  "V_FV2"
  Demux20/1 -> V_6/1, To Workspace20/1  "V_6"
  [IabcLL_Bus_3] -> Demux31/1
  [Iabc_B1_PV] -> Demux3/1
  [VabcLL_Bus_9] -> Demux12/1
  Demux5/1 -> Scope5/1, To Workspace4/1  "I_a_B1DC1"
  Demux14/1 -> Scope16/1, To Workspace14/1  "V_10"
  [Iabc_B1_busDC2] -> Demux7/1
  Demux21/1 -> Scope23/1, To Workspace21/1  "I_6"
  [VabcLL_Bus_8] -> Demux10/1
  Demux27/1 -> Scope29/1, To Workspace27/1  "I_2"
  Demux13/1 -> Scope15/1, To Workspace13/1  "I_9"
  [VabcLL_Bus_10] -> Demux14/1
  [IabcLL_Bus_4] -> Demux25/1
  [VabcLL_Bus_4] -> Demux24/1
  [IabcLL_Bus_5] -> Demux23/1
  Demux11/1 -> Scope13/1, To Workspace11/1  "I_8"
  [IabcLL_Bus_9] -> Demux13/1
  [IabcLL_Bus_2] -> Demux27/1
  [VabcLL_Bus_5] -> Demux22/1
  Demux15/1 -> Scope17/1, To Workspace15/1  "I_10"
  Demux3/1 -> Scope2/1, To Workspace3/1  "I_FV2"
  Demux16/1 -> Scope18/1, To Workspace16/1  "V_11"
  [IabcLL_Bus_14] -> Demux33/1
  Demux24/1 -> V_4/1, To Workspace24/1  "V_4"
  [VabcLL_Bus_14] -> Demux32/1
  [Iabc_Sec] -> Demux9/1
  Demux6/1 -> Scope6/1, To Workspace7/1  "V_a_B1DC2"
  [IabcLL_Bus_11] -> Demux17/1
  Demux1/1 -> Scope9/1, To Workspace1/1  "I_7"
  Demux23/1 -> Scope25/1, To Workspace23/1  "I_5"
  Demux29/1 -> Scope11/1, To Workspace29/1  "I_1"
  [Iabc_B1_busDC1] -> Demux5/1
  [IabcLL_Bus_8] -> Demux11/1
  Demux26/1 -> Scope28/1, To Workspace26/1  "V_2"
  [VabcLL_Bus_12] -> Demux18/1
  Demux19/1 -> Scope21/1, To Workspace19/1  "I_12"
  Demux28/1 -> Scope10/1, To Workspace28/1  "V_1"
  Demux17/1 -> Scope19/1, To Workspace17/1  "I_11"
  Demux33/1 -> Scope34/1, To Workspace33/1  "I_14"
  [VabcLL_Bus_6] -> Demux20/1
  [VabcLL_Bus_2] -> Demux26/1
  Demux10/1 -> Scope12/1, To Workspace10/1  "V_8"
  [VabcLL_Bus_11] -> Demux16/1
  Demux32/1 -> Scope33/1, To Workspace32/1  "V_14"
  Demux/1 -> V_7/1, To Workspace/1  "V_7"
  Demux25/1 -> Scope27/1, To Workspace25/1  "I_4"
  Demux30/1 -> Scope30/1, To Workspace30/1  "V_3"
  Demux31/1 -> Scope31/1, To Workspace31/1  "I_3"
  Demux4/1 -> Scope4/1, To Workspace5/1  "V_a_B1DC1"
  [Vabc_B1_PV] -> Demux2/1
  Demux8/1 -> V_a_red/1, To Workspace8/1  "V_a_red"
  [IabcLL_Bus_1] -> Demux29/1
  Demux22/1 -> V_5/1, To Workspace22/1  "V_5"
  Demux9/1 -> I_a_red/1, To Workspace9/1  "I_a_red"
  [IabcLL_Bus_6] -> Demux21/1
  [IabcLL_Bus_7] -> Demux1/1
  [Vabc_Sec] -> Demux8/1
  [Vabc_B575] -> Demux35/1  "Vabc_B575 (pu)"
  [Iabc_B575] -> Demux34/1  "Vabc_B575 (pu)"
  Demux35/1 -> Va_B575 (pu)/1  "Va_B575 (pu)"
  Demux34/1 -> Ia_B575 (pu)/1  "Ia_B575 (pu)"
  Demux36/1 -> Ia_B575/1  "Ia_B575"
  Demux37/1 -> Va_B575/1  "Va_B575"
  [Iabc_Aero] -> Demux36/1  "Iabc_B575"
  [Vabc_Aero] -> Demux37/1  "Vabc_B575"
  [Vabc_B13kv] -> Demux39/1  "Vabc_B13kv"
  [Iabc_B13kv] -> Demux38/1  "Iabc_B13kv"
  Demux39/1 -> Va_B13kv/1  "Va_B13kv"
  Demux38/1 -> Ia_B13kv/1  "Ia_B13kv"

== system Model_14Bus_Microgrid_paper_Latam/Red principal ==
  Primario (69 kV) : spsThreePhaseVIMeasurementLib/Three-Phase V-I Measurement  VoltageMeasurement=phase-to-ground  SetLabelV=on  LabelV=Vabc_Prim_pu  Vpu=off  VpuLL=on  CurrentMeasurement=yes  SetLabelI=on  LabelI=Iabc_Prim  Ipu=on  Pbase=100e6  Vbase=69e3/sqrt(2)  OutputType=Magnitude  PhasorSimulation=off  PSBequivalent=0
  Red principal 69 kV : Subsystem
      mask Display: image('/Users/christian/Documents/MATLAB/doctorado/4 conectada a la red con generador diesel, con generacion renovanble (fv)-con almacenamiento varios scope/Icons/Main-grid.png'); % Use "Edit Image" on toolstrip to change.
  Secundario 13.8 kV LL : spsThreePhaseVIMeasurementLib/Three-Phase V-I Measurement  VoltageMeasurement=phase-to-phase  SetLabelV=on  LabelV=Vabc_Sec_pu  Vpu=off  VpuLL=on  CurrentMeasurement=yes  SetLabelI=on  LabelI=Iabc_Sec_pu  Ipu=off  Pbase=250e6  Vbase=Vnom_prim/sqrt(2)  OutputType=Magnitude  PhasorSimulation=off  PSBequivalent=0
  Transformador (T3) 69kV / 13.8 kV 4 MVA : spsThreePhaseTransformerTwoWindingsLib/Three-Phase Transformer (Two Windings)  Winding1Connection=Yg  Winding2Connection=Delta (D1)  CoreType=Three single-phase transformers  SetSaturation=off  Hysteresis=off  DataFile='hysteresis'  SetInitialFlux=off  Measurements=None  UNITS=pu  NominalPower=[Pnom_T3 , Fnom ]  Winding1=[V1_LL_T3 , 0.015/2 , 0.015/(2*377)]  Winding2=[ Vnom_prim, 0.015/2 , 0.015/(2*377)]  Rm=500  Lm=500  L0=0.5  Saturation="[ 0,0  ;  0.005,1.2  ;  1.0,1.4 ]"  InitialFluxes=[ 0.8 , -0.8 , 0.7 ]  BreakLoop=off  DiscreteSolver=Trapezoidal iterative  DataType=off  TransfoNumber=0
  a : PMIOPort  Side=Left
  b : PMIOPort  Port=2  Side=Left
  c : PMIOPort  Port=3  Side=Left
  connections:
  Primario (69 kV)/RConn1 -- Transformador (T3) 69kV / 13.8 kV 4 MVA/LConn1
  Primario (69 kV)/RConn2 -- Transformador (T3) 69kV / 13.8 kV 4 MVA/LConn2
  Primario (69 kV)/LConn3 -- Red principal 69 kV/RConn1
  Primario (69 kV)/LConn1 -- Red principal 69 kV/RConn3
  Secundario 13.8 kV LL/RConn1 -- a/RConn1
  Secundario 13.8 kV LL/RConn2 -- b/RConn1
  Transformador (T3) 69kV / 13.8 kV 4 MVA/RConn1 -- Secundario 13.8 kV LL/LConn1
  Secundario 13.8 kV LL/RConn3 -- c/RConn1
  Transformador (T3) 69kV / 13.8 kV 4 MVA/RConn2 -- Secundario 13.8 kV LL/LConn2
  Primario (69 kV)/LConn2 -- Red principal 69 kV/RConn2
  Transformador (T3) 69kV / 13.8 kV 4 MVA/RConn3 -- Secundario 13.8 kV LL/LConn3
  Primario (69 kV)/RConn3 -- Transformador (T3) 69kV / 13.8 kV 4 MVA/LConn3

== system Model_14Bus_Microgrid_paper_Latam/Solar PV  ==
  note: ---------------
  note: DC Bus
  note: -
  note: +
  note: 725 kW
  note: AC Bus
  note: ---------------
  "  Sistema PV " : Subsystem
      mask Display: image('/Users/christian/Documents/MATLAB/doctorado/4 conectada a la red con generador diesel, con generacion renovanble (fv)-con almacenamiento varios scope/Icons/PV.png'); % Use "Edit Image" on toolstrip to change.
  "Inversor PV 480 / 250 DC / AC " : Subsystem
      mask Display: image('/Users/christian/Documents/MATLAB/doctorado/4 conectada a la red con generador diesel, con generacion renovanble (fv)-con almacenamiento varios scope/Icons/Inverter.png'); % Use "Edit Image" on toolstrip to change.
  Recurso solar : Subsystem
      mask Display: image('/Users/christian/Documents/MATLAB/doctorado/4 conectada a la red con generador diesel, con generacion renovanble (fv)-con almacenamiento varios scope/Icons/R_Sol.jpg'); % Use "Edit Image" on toolstrip to change.
  TPV 13.8 KV / 250 V 1 MVA : spsThreePhaseTransformerTwoWindingsLib/Three-Phase Transformer (Two Windings)  Winding1Connection=Yg  Winding2Connection=Delta (D1)  CoreType=Three single-phase transformers  SetSaturation=off  Hysteresis=off  DataFile='hysteresis'  SetInitialFlux=off  Measurements=None  UNITS=pu  NominalPower=[Pnom_xfo, Fnom ]  Winding1=W1_xfo  Winding2=W2_xfo  Rm=Rm_xfo  Lm=Lm_xfo  L0=0.5  Saturation=[ 0,0 ; 0.0024,1.2 ; 1.0,1.52 ]  InitialFluxes=[ 0.8 , -0.8 , 0.7 ]  BreakLoop=off  DiscreteSolver=Trapezoidal iterative  DataType=off  TransfoNumber=0
  A : PMIOPort  Side=Right
  B : PMIOPort  Port=2  Side=Right
  C : PMIOPort  Port=3  Side=Right
  wires:
  Recurso solar/2(temp) -> "  Sistema PV "/2(Temp2)
  Recurso solar/1(Ir2) -> "  Sistema PV "/1(Irradiance)
  connections:
  TPV 13.8 KV / 250 V 1 MVA/LConn1 -- A/RConn1
  TPV 13.8 KV / 250 V 1 MVA/LConn3 -- C/RConn1
  B/RConn1 -- TPV 13.8 KV / 250 V 1 MVA/LConn2
  TPV 13.8 KV / 250 V 1 MVA/RConn2 -- "Inversor PV 480 / 250 DC / AC "/RConn2
  TPV 13.8 KV / 250 V 1 MVA/RConn1 -- "Inversor PV 480 / 250 DC / AC "/RConn1
  "Inversor PV 480 / 250 DC / AC "/RConn3 -- TPV 13.8 KV / 250 V 1 MVA/RConn3
  "  Sistema PV "/LConn2 -- "Inversor PV 480 / 250 DC / AC "/LConn2
  "  Sistema PV "/LConn1 -- "Inversor PV 480 / 250 DC / AC "/LConn1

== system Model_14Bus_Microgrid_paper_Latam/Subsystem1 ==
  note: ---------------
  note: Bus AC
  note: +
  note: -
  Breaker bus DC1 : spsThreePhaseBreakerLib/Three-Phase Breaker  InitialState=closed  SwitchA=on  SwitchB=on  SwitchC=on  SwitchTimes="[4/60  10/60]"  External=on  BreakerResistance=0.001  SnubberResistance=1e6  SnubberCapacitance=inf  Measurements=None
  Bus AC / DC 1 : spsThreePhaseVIMeasurementLib/Three-Phase V-I Measurement  VoltageMeasurement=phase-to-ground  SetLabelV=on  LabelV=Vabc_B1_busDC1  Vpu=off  VpuLL=off  CurrentMeasurement=yes  SetLabelI=on  LabelI=Iabc_B1_busDC1  Ipu=off  Pbase=100e6  Vbase=25e3  OutputType=Complex  PhasorSimulation=off  PSBequivalent=0
  Bus_AC/DC4 : Subsystem
  Control measurement : Subsystem
  Convertidor bidireccional 1.1 300 (DC) / 150 V (AC) P_nom 3kW : Subsystem
      mask Display: image('/Users/christian/Documents/MATLAB/doctorado/4 conectada a la red con generador diesel, con generacion renovanble (fv)-con almacenamiento varios scope/Icons/Bi-directional converter.png'); % Use "Edit Image" on toolstrip to change.
  On/off grid bus DC1 : Constant
  "                                          A" : PMIOPort  Side=Left
  "                                          B" : PMIOPort  Port=2  Side=Left
  "                                          C" : PMIOPort  Port=3  Side=Left
  B1 - : PMIOPort  Port=4  Side=Right
  B1 + : PMIOPort  Port=5  Side=Right
  tag scope: Means=global
  wires:
  [Means] -> Convertidor bidireccional 1.1 300 (DC) / 150 V (AC) P_nom 3kW/1(Means)
  Control measurement/1("              Out1") -> [Means]
  On/off grid bus DC1/1 -> Breaker bus DC1/1
  connections:
  Bus AC / DC 1/RConn2 -- Breaker bus DC1/LConn2
  Breaker bus DC1/RConn2 -- "                                          B"/RConn1 -- Control measurement/LConn2
  Breaker bus DC1/RConn1 -- "                                          A"/RConn1 -- Control measurement/LConn3
  Convertidor bidireccional 1.1 300 (DC) / 150 V (AC) P_nom 3kW/RConn2 -- B1 -/RConn1
  Bus AC / DC 1/LConn3 -- Convertidor bidireccional 1.1 300 (DC) / 150 V (AC) P_nom 3kW/LConn3
  Bus AC / DC 1/LConn2 -- Convertidor bidireccional 1.1 300 (DC) / 150 V (AC) P_nom 3kW/LConn2
  Bus AC / DC 1/LConn1 -- Convertidor bidireccional 1.1 300 (DC) / 150 V (AC) P_nom 3kW/LConn1
  Bus AC / DC 1/RConn3 -- Breaker bus DC1/LConn3
  Bus AC / DC 1/RConn1 -- Breaker bus DC1/LConn1
  Breaker bus DC1/RConn3 -- "                                          C"/RConn1 -- Control measurement/LConn1
  Convertidor bidireccional 1.1 300 (DC) / 150 V (AC) P_nom 3kW/RConn1 -- B1 +/RConn1

== system Model_14Bus_Microgrid_paper_Latam/Subsystem2 ==
  note: 320 kVA ; cos (phi) = 1
  Breaker Load 9 : spsThreePhaseBreakerLib/Three-Phase Breaker  InitialState=closed  SwitchA=on  SwitchB=on  SwitchC=on  SwitchTimes="[4/60  10/60]"  External=on  BreakerResistance=0.001  SnubberResistance=1e6  SnubberCapacitance=inf  Measurements=None
  Non Linear AC  Load 9 : Subsystem
      mask Display: image('/Users/christian/Documents/MATLAB/doctorado/4 conectada a la red con generador diesel, con generacion renovanble (fv)-con almacenamiento varios scope/Icons/horno_de_arco.png'); % Use "Edit Image" on toolstrip to change.
  On/off Load 9 : Constant
  A : PMIOPort  Side=Left
  B : PMIOPort  Port=2  Side=Left
  C : PMIOPort  Port=3  Side=Left
  wires:
  On/off Load 9/1 -> Breaker Load 9/1
  connections:
  B/RConn1 -- Breaker Load 9/LConn2
  Breaker Load 9/LConn1 -- A/RConn1
  Non Linear AC  Load 9/LConn2 -- Breaker Load 9/RConn2
  C/RConn1 -- Breaker Load 9/LConn3
  Non Linear AC  Load 9/LConn3 -- Breaker Load 9/RConn3
  Non Linear AC  Load 9/LConn1 -- Breaker Load 9/RConn1

== system Model_14Bus_Microgrid_paper_Latam/Subsystem3 ==
  note: -
  note: +
  note: ---------------
  note: Bus AC
  Breaker bus DC2 : spsThreePhaseBreakerLib/Three-Phase Breaker  InitialState=closed  SwitchA=on  SwitchB=on  SwitchC=on  SwitchTimes="[4/60  10/60]"  External=on  BreakerResistance=0.001  SnubberResistance=1e6  SnubberCapacitance=inf  Measurements=None
  Bus AC / DC 2 : spsThreePhaseVIMeasurementLib/Three-Phase V-I Measurement  VoltageMeasurement=phase-to-ground  SetLabelV=on  LabelV=Vabc_B1_busDC2  Vpu=off  VpuLL=off  CurrentMeasurement=yes  SetLabelI=on  LabelI=Iabc_B1_busDC2  Ipu=off  Pbase=100e6  Vbase=25e3  OutputType=Complex  PhasorSimulation=off  PSBequivalent=0
  Bus_AC/DC5 : Subsystem
  Control measurement2 : Subsystem
  Convertidor bidireccional 1.2 300 (DC) / 150 V (AC) P_nom 3kW : Subsystem
      mask Display: image('/Users/christian/Documents/MATLAB/doctorado/4 conectada a la red con generador diesel, con generacion renovanble (fv)-con almacenamiento varios scope/Icons/Bi-directional converter.png'); % Use "Edit Image" on toolstrip to change.
  On/off grid bus DC2 OP_max / min1 : Subsystem
  a : PMIOPort  Side=Left
  b : PMIOPort  Port=2  Side=Left
  "                                          C" : PMIOPort  Port=3  Side=Left
  B1 + : PMIOPort  Port=4  Side=Left
  B1 - : PMIOPort  Port=5  Side=Left
  tag scope: Means2=global
  wires:
  [Means2] -> Convertidor bidireccional 1.2 300 (DC) / 150 V (AC) P_nom 3kW/1(Means2)
  Control measurement2/1("              Out1") -> [Means2]
  On/off grid bus DC2 OP_max / min1/1(on / off) -> Breaker bus DC2/1
  connections:
  Convertidor bidireccional 1.2 300 (DC) / 150 V (AC) P_nom 3kW/RConn1 -- B1 +/RConn1
  Convertidor bidireccional 1.2 300 (DC) / 150 V (AC) P_nom 3kW/RConn2 -- B1 -/RConn1
  Bus AC / DC 2/LConn3 -- Convertidor bidireccional 1.2 300 (DC) / 150 V (AC) P_nom 3kW/LConn3
  Bus AC / DC 2/RConn3 -- Breaker bus DC2/LConn3
  Control measurement2/LConn3 -- a/RConn1 -- Breaker bus DC2/RConn1
  Bus AC / DC 2/LConn1 -- Convertidor bidireccional 1.2 300 (DC) / 150 V (AC) P_nom 3kW/LConn1
  Bus AC / DC 2/RConn1 -- Breaker bus DC2/LConn1
  Bus AC / DC 2/LConn2 -- Convertidor bidireccional 1.2 300 (DC) / 150 V (AC) P_nom 3kW/LConn2
  Control measurement2/LConn2 -- b/RConn1 -- Breaker bus DC2/RConn2
  Breaker bus DC2/RConn3 -- "                                          C"/RConn1 -- Control measurement2/LConn1
  Bus AC / DC 2/RConn2 -- Breaker bus DC2/LConn2

== system Model_14Bus_Microgrid_paper_Latam/Subsystem4 ==
  Breaker2 : spsBreakerLib/Breaker  InitialState=1  SwitchingTimes="[1/60  5/60]"  External=on  BreakerResistance=0.01  SnubberResistance=1e6  SnubberCapacitance=inf  Measurements=None  MoreParameters=on  NoBreakLoop=off
  Breaker3 : spsBreakerLib/Breaker  InitialState=1  SwitchingTimes="[1/60  5/60]"  External=on  BreakerResistance=0.01  SnubberResistance=1e6  SnubberCapacitance=inf  Measurements=None  MoreParameters=on  NoBreakLoop=off
  OP_max / min : Subsystem
  Subsystem5 : Subsystem
  4 : PMIOPort  Side=Left
  3 : PMIOPort  Port=2  Side=Left
  1 : PMIOPort  Port=3  Side=Right
  2 : PMIOPort  Port=4  Side=Right
  wires:
  OP_max / min/1(on / off) -> Breaker3/1, Breaker2/1
  connections:
  2/RConn1 -- Breaker2/RConn1
  1/RConn1 -- Breaker3/RConn1
  Subsystem5/RConn1 -- 4/RConn1 -- Breaker2/LConn1
  Subsystem5/RConn2 -- 3/RConn1 -- Breaker3/LConn1

== system Model_14Bus_Microgrid_paper_Latam/Adquisición de datos/Delta_abc ==
  Mux3 : Mux  Inputs=14
  f3 : ToWorkspace  VariableName=ang_abc  SaveFormat=Timeseries  SampleTime=-1
  wires:
  [delta_abc_Bus10] -> Mux3/10
  [delta_abc_Bus4] -> Mux3/4
  [delta_abc_Bus7] -> Mux3/7
  [delta_abc_Bus8] -> Mux3/8
  [delta_abc_Bus11] -> Mux3/11
  [delta_abc_Bus5] -> Mux3/5
  [delta_abc_Bus9] -> Mux3/9
  [delta_abc_Bus2] -> Mux3/2
  [delta_abc_Bus1] -> Mux3/1
  [delta_abc_Bus12] -> Mux3/12
  [delta_abc_Bus14] -> Mux3/14
  Mux3/1 -> f3/1
  [delta_abc_Bus6] -> Mux3/6
  [delta_abc_Bus13] -> Mux3/13
  [delta_abc_Bus3] -> Mux3/3

== system Model_14Bus_Microgrid_paper_Latam/Adquisición de datos/PF_abc ==
  Mux2 : Mux  Inputs=14
  f3 : ToWorkspace  VariableName=PF_abc  SaveFormat=Timeseries  SampleTime=-1
  wires:
  [PFabc_Bus2] -> Mux2/2
  [PFabc_Bus4] -> Mux2/4
  [PFabc_Bus1] -> Mux2/1
  [PFabc_Bus6] -> Mux2/6
  Mux2/1 -> f3/1
  [PFabc_Bus5] -> Mux2/5
  [PFabc_Bus14] -> Mux2/14
  [PFabc_Bus8] -> Mux2/8
  [PFabc_Bus9] -> Mux2/9
  [PFabc_Bus7] -> Mux2/7
  [PFabc_Bus11] -> Mux2/11
  [PFabc_Bus13] -> Mux2/13
  [PFabc_Bus10] -> Mux2/10
  [PFabc_Bus3] -> Mux2/3
  [PFabc_Bus12] -> Mux2/12

== system Model_14Bus_Microgrid_paper_Latam/Adquisición de datos/P_abc ==
  Mux : Mux  Inputs=15
  f1 : ToWorkspace  VariableName=P_abc  SaveFormat=Timeseries  SampleTime=-1
  wires:
  [P_abc_Bus1] -> Mux/1
  [P_abc_Bus3] -> Mux/3
  [P_abc_Bus2] -> Mux/2
  [P_abc_Bus13] -> Mux/13
  Mux/1 -> f1/1
  [P_abc_Bus12] -> Mux/12
  [P_abc_Bus9] -> Mux/9
  [P_abc_Bus8] -> Mux/8
  [P_abc_Bus10] -> Mux/10
  [P_abc_Bus11] -> Mux/11
  [P_abc_Bus7] -> Mux/7
  [P_abc_Bus4] -> Mux/4
  [P_abc_Bus14] -> Mux/14
  [P_abc_Bus5] -> Mux/5
  [P_BusDC] -> Mux/15
  [P_abc_Bus6] -> Mux/6

== system Model_14Bus_Microgrid_paper_Latam/Adquisición de datos/Power_Losses_abc ==
  Mux : Mux  Inputs=14
  f2 : ToWorkspace  VariableName=Power_Losse_abc  SaveFormat=Timeseries  SampleTime=-1
  wires:
  [Power_Losse_abc_L12] -> Mux/12
  [Power_Losse_abc_L10] -> Mux/10
  [Power_Losse_abc_L13] -> Mux/13
  [Power_Losse_abc_L1] -> Mux/1
  Mux/1 -> f2/1
  [Power_Losse_abc_L2] -> Mux/2
  [Power_Losse_abc_L3] -> Mux/3
  [Power_Losse_abc_L4] -> Mux/4
  [Power_Losse_abc_L5] -> Mux/5
  [Power_Losse_abc_L14] -> Mux/14
  [Power_Losse_abc_L9] -> Mux/9
  [Power_Losse_abc_L6] -> Mux/6
  [Power_Losse_abc_L8] -> Mux/8
  [Power_Losse_abc_L11] -> Mux/11
  [Power_Losse_abc_L7] -> Mux/7

== system Model_14Bus_Microgrid_paper_Latam/Adquisición de datos/Q_abc ==
  Mux2 : Mux  Inputs=14
  f2 : ToWorkspace  VariableName=Q_abc  SaveFormat=Timeseries  SampleTime=-1
  wires:
  Mux2/1 -> f2/1
  [Q_abc_Bus6] -> Mux2/6
  [Q_abc_Bus1] -> Mux2/1
  [Q_abc_Bus4] -> Mux2/4
  [Q_abc_Bus5] -> Mux2/5
  [Q_abc_Bus9] -> Mux2/9
  [Q_abc_Bus10] -> Mux2/10
  [Q_abc_Bus2] -> Mux2/2
  [Q_abc_Bus12] -> Mux2/12
  [Q_abc_Bus8] -> Mux2/8
  [Q_abc_Bus13] -> Mux2/13
  [Q_abc_Bus3] -> Mux2/3
  [Q_abc_Bus11] -> Mux2/11
  [Q_abc_Bus14] -> Mux2/14
  [Q_abc_Bus7] -> Mux2/7

== system Model_14Bus_Microgrid_paper_Latam/Adquisición de datos/THDi_abc ==
  Mux1 : Mux  Inputs=14
  f1 : ToWorkspace  VariableName=THDi_abc  SaveFormat=Timeseries  SampleTime=-1
  wires:
  [THDi_abc_Bus12] -> Mux1/12
  [THDi_abc_Bus10] -> Mux1/10
  [THDi_abc_Bus13] -> Mux1/13
  [THDi_abc_Bus2] -> Mux1/2
  [THDi_abc_Bus3] -> Mux1/3
  [THDi_abc_Bus14] -> Mux1/14
  [THDi_abc_Bus6] -> Mux1/6
  [THDi_abc_Bus9] -> Mux1/9
  [THDi_abc_Bus4] -> Mux1/4
  [THDi_abc_Bus11] -> Mux1/11
  [THDi_abc_Bus7] -> Mux1/7
  Mux1/1 -> f1/1
  [THDi_abc_Bus1] -> Mux1/1
  [THDi_abc_Bus5] -> Mux1/5
  [THDi_abc_Bus8] -> Mux1/8

== system Model_14Bus_Microgrid_paper_Latam/Adquisición de datos/THDv_abc ==
  Mux1 : Mux  Inputs=14
  f1 : ToWorkspace  VariableName=THDv_abc  SaveFormat=Timeseries  SampleTime=-1
  wires:
  [THDv_abc_Bus8] -> Mux1/8
  [THDv_abc_Bus5] -> Mux1/5
  [THDv_abc_Bus1] -> Mux1/1
  Mux1/1 -> f1/1
  [THDv_abc_Bus7] -> Mux1/7
  [THDv_abc_Bus11] -> Mux1/11
  [THDv_abc_Bus4] -> Mux1/4
  [THDv_abc_Bus9] -> Mux1/9
  [THDv_abc_Bus6] -> Mux1/6
  [THDv_abc_Bus14] -> Mux1/14
  [THDv_abc_Bus3] -> Mux1/3
  [THDv_abc_Bus2] -> Mux1/2
  [THDv_abc_Bus13] -> Mux1/13
  [THDv_abc_Bus10] -> Mux1/10
  [THDv_abc_Bus12] -> Mux1/12

== system Model_14Bus_Microgrid_paper_Latam/Adquisición de datos/VoltageLL_pu_abc ==
  Mux : Mux  Inputs=15
  f2 : ToWorkspace  VariableName=VoltageLL_pu_abc  SaveFormat=Timeseries  SampleTime=-1
  wires:
  [Vabc_LL_pu_Bus4] -> Mux/4
  [Vabc_LL_pu_Bus3] -> Mux/3
  [Vabc_LL_pu_Bus5] -> Mux/5
  Mux/1 -> f2/1
  [Vabc_LL_pu_Bus8] -> Mux/8
  [Vabc_LL_pu_Bus1] -> Mux/1
  [Vabc_LL_pu_Bus2] -> Mux/2
  [Vabc_LL_pu_Bus11] -> Mux/11
  [Vabc_LL_pu_Bus12] -> Mux/12
  [Vabc_LL_pu_Bus6] -> Mux/6
  [Vabc_LL_pu_Bus14] -> Mux/14
  [Vabc_LL_pu_Bus7] -> Mux/7
  [V_pu_BusDC] -> Mux/15
  [Vabc_LL_pu_Bus13] -> Mux/13
  [Vabc_LL_pu_Bus9] -> Mux/9
  [Vabc_LL_pu_Bus10] -> Mux/10
